simulink model "Amp_baseline1"  (R2020a)
settings: Solver=ode45  StartTime=0.0  StopTime=60  RelTol=1e-3
model workspace (MAT data in the model file):
  WinSize = Simulink.Parameter
  WinSize.Value = 16
  WinSize.DataType = 'double'
  WinSize.Dimensions = [1 1]
  cfg_native : object (value not decoded)
  en_add_channels = 1
  fc_bandpass = Simulink.Parameter
  fc_bandpass.Value = [0.05 0.26]
  fc_bandpass.DataType = 'double'
  fc_bandpass.Dimensions = [1 2]
  host_ip = 2130706433
  host_port = 50223
  local_ip = 2130706433
  local_port = 50224
  num_en_channels = 32
  num_samples = 1
  sample_rate = 250
  serial_number = 'NB-2015.10.93'
undefined symbols (not defined in the file or in its folder): currentCFG_Amp_baseline_UB, UB
libraries: gtecHighspeedLib x17, TobiiEyeTrackerLib x1, gUSBamplib x1
settings Model: ModifiedByFormat=g.tec  Creator=g.tec medical engineering  LastModifiedBy=g.tec
settings DataIOCC: LimitDataPoints=on  SaveFormat=Array  ReturnWorkspaceOutputs=off
settings OptimizationCC: BlockReduction=off  BooleanDataType=off  LifeSpan=inf
settings DebuggingCC: SaveWithParameterizedLinksMsg=none  UnderspecifiedInitializationDetection=Classic  MergeDetectMultiDrivingBlocksExec=none  SignalResolutionControl=TryResolveAllWithWarning  FrameProcessingCompatibilityMsg=none  SFUnexpectedBacktrackingDiag=warning  SFNoUnconditionalDefaultTransitionDiag=warning  SFExecutionAtInitializationDiag=none  ArithmeticOperatorsInVariantConditions=warning
settings HardwareCC: ProdBitPerPointer=32  ProdBitPerSizeT=32  ProdBitPerPtrDiffT=32  ProdLargestAtomicFloat=None  ProdIntDivRoundTo=Undefined  ProdEndianess=Unspecified  ProdWordSize=32  ProdHWDeviceType=32-bit Generic  TargetUnknown=on
settings ModelReferenceCC: PropagateSignalLabelsOutOfModel=off
settings SFSimCC: SimUseLocalCustomCode=off  CustomCodeUndefinedFunction=UseInterfaceOnly
settings RTWCC: RTWUseLocalCustomCode=off
settings CodeAppCC: StateflowObjectComments=on
settings GRTTargetCC: TargetLangStandard=C89/C90 (ANSI)
settings ConfigComp: CovMetricSettings=dw  CovHtmlReporting=on  CovSaveCumulativeToWorkspaceVar=on  CovSaveSingleToWorkspaceVar=on  CovExternalEMLEnable=off

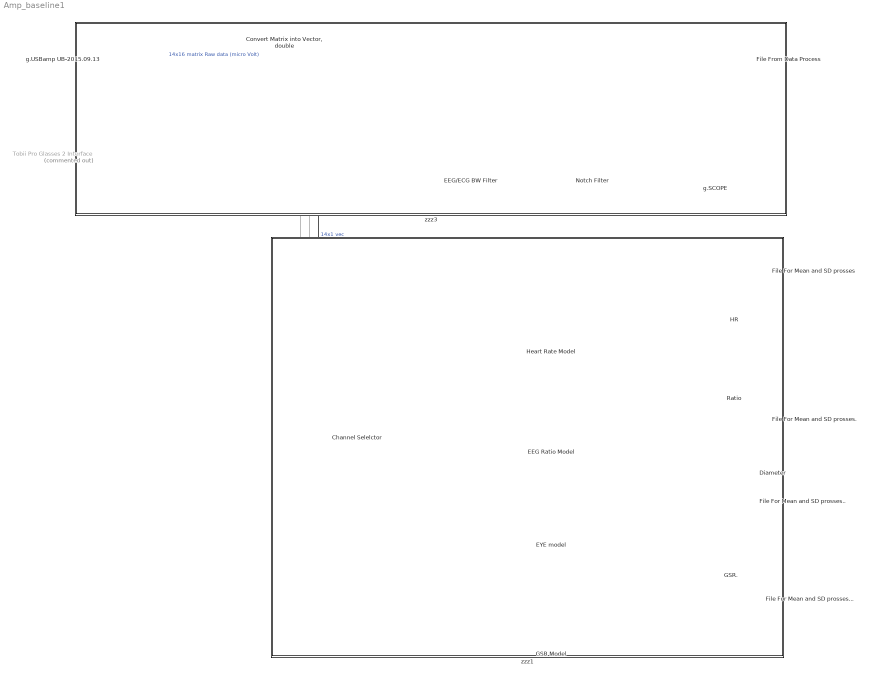
== system Amp_baseline1 ==
  Channel Selelctor : Subsystem
  "Convert Matrix into Vector, double" : Subsystem
  Diameter : Display
  EEG Ratio Model : Subsystem  ReferencedSubsystem=EEG_Ratio_Model
  EEG/ECG BW Filter : gtecHighspeedLib/EEG//ECG BW Filter  Order=6  LowerFreq=0.1  UpperFreq=30  SampFreq=512
      settings: SourceProductName=g.HIsys Library
  EYE model : Subsystem  ReferencedSubsystem=Pupil_Diameter_Model_BaseLine
  File For Mean and SD prosses : ToFile  Filename=HeartRate.mat  MatrixName=heartRatedata
  File For Mean and SD prosses. : ToFile  Filename=Ratio.mat  MatrixName=Ratio
  File For Mean and SD prosses.. : ToFile  Filename=Eye_Diameter.mat  MatrixName=Eye_Diameter
  File For Mean and SD prosses... : ToFile  Filename=GSR.mat  MatrixName=GSR
  File From Data Process : ToFile  Filename=Baseline.mat  MatrixName=Baselinedata
  GSR Model : Subsystem  ReferencedSubsystem=GSR_Model
  GSR. : Display
  HR : Display
  Heart Rate Model : Subsystem  ReferencedSubsystem=Heart_Rate_Model
  Notch Filter : gtecHighspeedLib/Notch Filter  Order=2  NotchFreq=50  SampFreq=512
      settings: SourceProductName=g.tec Highspeed Library
  Ratio : Display
  Tobii Pro Glasses 2 Interface : TobiiEyeTrackerLib/Tobii Pro Glasses 2 Interface  Commented=on  Key=0  pc_right=off  pc_left=off  pd_right=off  pd_left=off  gd_right=off  gd_left=off  gp=on  gp3=off  gy=off  ac=off
      settings: SourceProductName=g.EYEtracking Interface (Tobii Pro Glasses 2)
  g.SCOPE : gtecHighspeedLib/g.SCOPE
      settings: SourceProductName=g.HIsys Library
  g.USBamp UB-2015.09.13 : gUSBamplib/g.USBamp  cfg=currentCFG_Amp_baseline_UB-2015.09.13.cfg  snr=UB-2015.09.13
      settings: SourceProductName=g.USBamp
  zzz1 : Subsystem  TreatAsAtomicUnit=on
      settings: OpenFcn=% no-op
      mask Display: disp('')
  zzz3 : Subsystem  TreatAsAtomicUnit=on
      settings: OpenFcn=% no-op
      mask Display: disp('')
  wires:
  g.USBamp UB-2015.09.13/1 -> "Convert Matrix into Vector, double"/1(In)  "14x16 matrix Raw data (micro Volt)"
  "Convert Matrix into Vector, double"/1(All channels) -> File From Data Process/1, EEG/ECG BW Filter/1, Channel Selelctor/1(14x1 vec)  "14x1 vec"
  EEG Ratio Model/1 -> File For Mean and SD prosses./1, Ratio/1
  Heart Rate Model/2 -> HR/1
  Heart Rate Model/1 -> File For Mean and SD prosses/1
  EYE model/1 -> Diameter/1, File For Mean and SD prosses../1
  GSR Model/1 -> GSR./1, File For Mean and SD prosses.../1
  Channel Selelctor/1(ECG) -> Heart Rate Model/1
  Channel Selelctor/13(GSR) -> GSR Model/1
  Channel Selelctor/2(EEG1) -> EEG Ratio Model/1
  Channel Selelctor/3(EEG2) -> EEG Ratio Model/2
  Channel Selelctor/4(EEG3) -> EEG Ratio Model/3
  Channel Selelctor/5(EEG4) -> EEG Ratio Model/4
  Channel Selelctor/6(EEG5) -> EEG Ratio Model/5
  Channel Selelctor/7(EEG6) -> EEG Ratio Model/6
  Channel Selelctor/8(EEG7) -> EEG Ratio Model/7
  Channel Selelctor/9(EEG8) -> EEG Ratio Model/8
  Channel Selelctor/10(EEG9) -> EEG Ratio Model/9
  Channel Selelctor/11(EEG10) -> EEG Ratio Model/10
  Channel Selelctor/12(EEG11) -> EEG Ratio Model/11
  Channel Selelctor/14(EEG12) -> EEG Ratio Model/12
  Tobii Pro Glasses 2 Interface/3 -> EYE model/2
  Tobii Pro Glasses 2 Interface/4 -> EYE model/1
  Notch Filter/1 -> g.SCOPE/1
  EEG/ECG BW Filter/1 -> Notch Filter/1

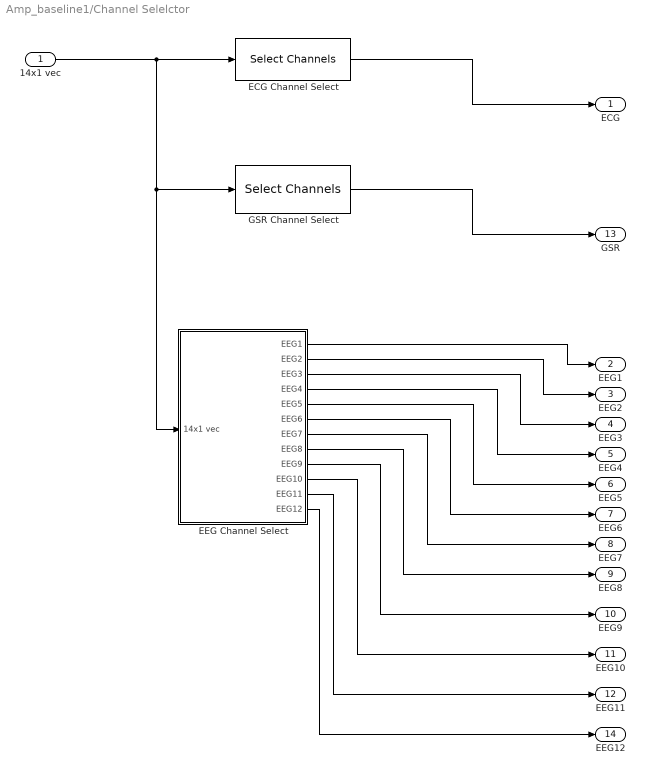
== system Amp_baseline1/Channel Selelctor ==
  14x1 vec : Inport
  ECG Channel Select : gtecHighspeedLib/Select Channels  selectedchannels=[2]  totalchannels=14
      settings: SourceProductName=g.HIsys Library
  EEG Channel Select : Subsystem
  GSR Channel Select : gtecHighspeedLib/Select Channels  selectedchannels=[1]  totalchannels=14
      settings: SourceProductName=g.HIsys Library
  ECG : Outport
  EEG1 : Outport  Port=2
  EEG2 : Outport  Port=3
  EEG3 : Outport  Port=4
  EEG4 : Outport  Port=5
  EEG5 : Outport  Port=6
  EEG6 : Outport  Port=7
  EEG7 : Outport  Port=8
  EEG8 : Outport  Port=9
  EEG9 : Outport  Port=10
  EEG10 : Outport  Port=11
  EEG11 : Outport  Port=12
  GSR : Outport  Port=13
  EEG12 : Outport  Port=14
  wires:
  14x1 vec/1 -> ECG Channel Select/1, GSR Channel Select/1, EEG Channel Select/1(14x1 vec)
  ECG Channel Select/1 -> ECG/1
  GSR Channel Select/1 -> GSR/1
  EEG Channel Select/1(EEG1) -> EEG1/1
  EEG Channel Select/2(EEG2) -> EEG2/1
  EEG Channel Select/3(EEG3) -> EEG3/1
  EEG Channel Select/4(EEG4) -> EEG4/1
  EEG Channel Select/5(EEG5) -> EEG5/1
  EEG Channel Select/6(EEG6) -> EEG6/1
  EEG Channel Select/7(EEG7) -> EEG7/1
  EEG Channel Select/8(EEG8) -> EEG8/1
  EEG Channel Select/9(EEG9) -> EEG9/1
  EEG Channel Select/10(EEG10) -> EEG10/1
  EEG Channel Select/11(EEG11) -> EEG11/1
  EEG Channel Select/12(EEG12) -> EEG12/1

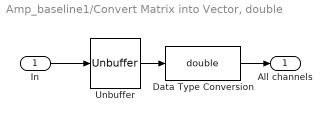
== system Amp_baseline1/Convert Matrix into Vector, double ==
  In : Inport
  Data Type Conversion : DataTypeConversion  OutDataTypeStr=double
  Unbuffer : Unbuffer
  All channels : Outport
  wires:
  In/1 -> Unbuffer/1
  Unbuffer/1 -> Data Type Conversion/1
  Data Type Conversion/1 -> All channels/1

== system Amp_baseline1/zzz1 ==

== system Amp_baseline1/zzz3 ==

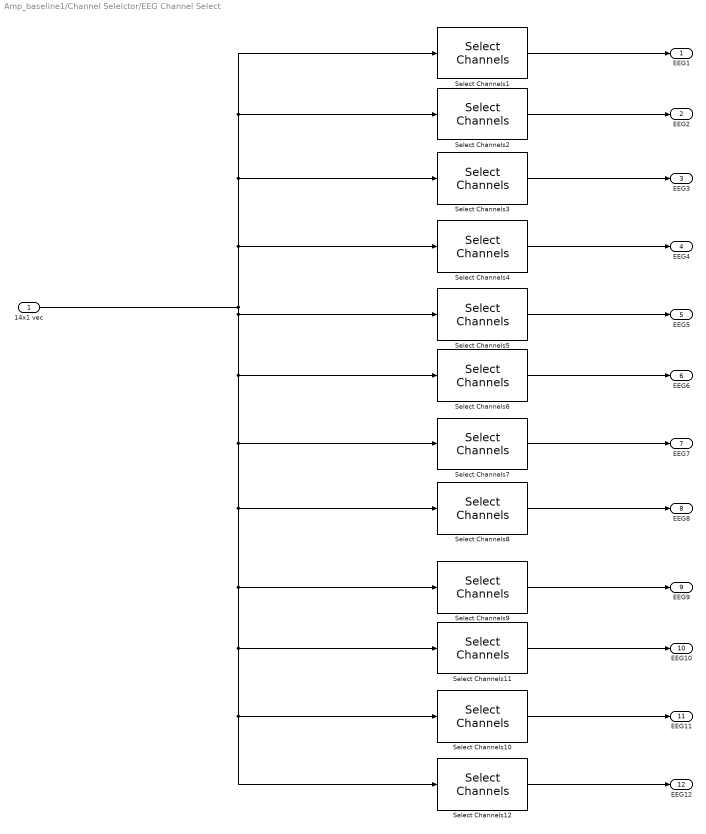
== system Amp_baseline1/Channel Selelctor/EEG Channel Select ==
  14x1 vec : Inport
  Select Channels1 : gtecHighspeedLib/Select Channels  selectedchannels=[3]  totalchannels=14
      settings: SourceProductName=g.HIsys Library
  Select Channels10 : gtecHighspeedLib/Select Channels  selectedchannels=[13]  totalchannels=14
      settings: SourceProductName=g.HIsys Library
  Select Channels11 : gtecHighspeedLib/Select Channels  selectedchannels=[12]  totalchannels=14
      settings: SourceProductName=g.HIsys Library
  Select Channels12 : gtecHighspeedLib/Select Channels  selectedchannels=[14]  totalchannels=14
      settings: SourceProductName=g.HIsys Library
  Select Channels2 : gtecHighspeedLib/Select Channels  selectedchannels=[4]  totalchannels=14
      settings: SourceProductName=g.HIsys Library
  Select Channels3 : gtecHighspeedLib/Select Channels  selectedchannels=[5]  totalchannels=14
      settings: SourceProductName=g.HIsys Library
  Select Channels4 : gtecHighspeedLib/Select Channels  selectedchannels=[6]  totalchannels=14
      settings: SourceProductName=g.HIsys Library
  Select Channels5 : gtecHighspeedLib/Select Channels  selectedchannels=[7]  totalchannels=14
      settings: SourceProductName=g.HIsys Library
  Select Channels6 : gtecHighspeedLib/Select Channels  selectedchannels=[8]  totalchannels=14
      settings: SourceProductName=g.HIsys Library
  Select Channels7 : gtecHighspeedLib/Select Channels  selectedchannels=[9]  totalchannels=14
      settings: SourceProductName=g.HIsys Library
  Select Channels8 : gtecHighspeedLib/Select Channels  selectedchannels=[10]  totalchannels=14
      settings: SourceProductName=g.HIsys Library
  Select Channels9 : gtecHighspeedLib/Select Channels  selectedchannels=[11]  totalchannels=14
      settings: SourceProductName=g.HIsys Library
  EEG1 : Outport
  EEG2 : Outport  Port=2
  EEG3 : Outport  Port=3
  EEG4 : Outport  Port=4
  EEG5 : Outport  Port=5
  EEG6 : Outport  Port=6
  EEG7 : Outport  Port=7
  EEG8 : Outport  Port=8
  EEG9 : Outport  Port=9
  EEG10 : Outport  Port=10
  EEG11 : Outport  Port=11
  EEG12 : Outport  Port=12
  wires:
  Select Channels7/1 -> EEG7/1
  Select Channels1/1 -> EEG1/1
  Select Channels8/1 -> EEG8/1
  Select Channels11/1 -> EEG10/1
  Select Channels2/1 -> EEG2/1
  Select Channels4/1 -> EEG4/1
  Select Channels5/1 -> EEG5/1
  Select Channels10/1 -> EEG11/1
  Select Channels9/1 -> EEG9/1
  Select Channels6/1 -> EEG6/1
  Select Channels3/1 -> EEG3/1
  14x1 vec/1 -> Select Channels8/1, Select Channels10/1, Select Channels12/1, Select Channels11/1, Select Channels9/1, Select Channels7/1, Select Channels6/1, Select Channels5/1, Select Channels4/1, Select Channels2/1, Select Channels1/1, Select Channels3/1
  Select Channels12/1 -> EEG12/1
